simulink model "Integrated_controlled_system"  (R2020a)
settings: Solver=VariableStepAuto  StartTime=0.0  StopTime=simStopTime  RelTol=1e-3
PostLoadFcn:
  | helperLFSetUp
values from neighbouring files (symbols this model uses):
  lr = 1.67    [LateralDynamicsCT05.m]    (also in controller_setup05.m; helperLFSetUp.m)
  m = 2272    [LateralDynamicsCT05.m]    (also in controller_setup05.m; helperLFSetUp.m)
  tau = 0.5    [helperLFSetUp.m]
  Tfault = 1    [helperLFSetUp.m]
  Ts = 0.1    [controller_setup05.m]    (also in helperLFSetUp.m)
  v_set = egoCar.v0    [helperLFSetUp.m]
undefined symbols (not defined in the file or in its folder): Curvature, CurvatureDerivative, driving, HeadingAngle, LateralOffset, Left, Right, Strength
libraries: drivingscenarioandsensors x5, autolibshared x1
CloseFcn:
  | helperLFCleanUp
settings Model: NumberOfSteps=10  Creator=The MathWorks, Inc.  LastModifiedBy=dekunw
settings DataIOCC: ReturnWorkspaceOutputs=off
settings DebuggingCC: ParameterPrecisionLossMsg=none  PregeneratedLibrarySubsystemCodeDiagnostic=none  ArithmeticOperatorsInVariantConditions=warning
settings HardwareCC: ProdLongLongMode=on
settings SFSimCC: SimUseLocalCustomCode=off
settings RTWCC: GenerateReport=on  RTWUseLocalCustomCode=off  LaunchReport=on
settings ConfigComp: CovScope=ReferencedModels  CovIncludeTopModel=off  CovHtmlReporting=on

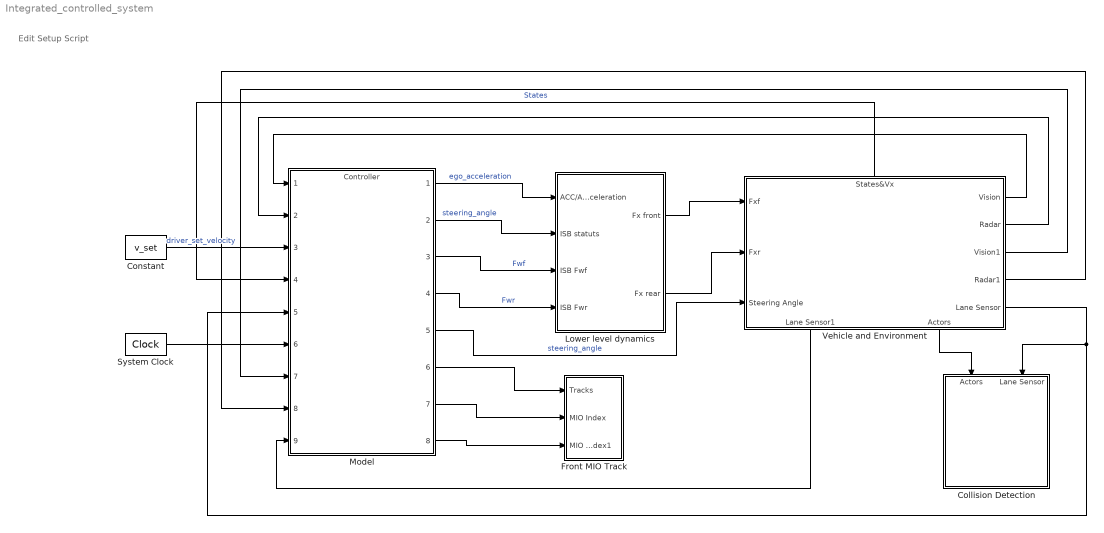
== system Integrated_controlled_system ==
  note: Edit Setup Script
  Collision Detection : Subsystem
  Constant : Constant  Value=v_set  SampleTime=Ts
  Front MIO Track : Subsystem
  Lower level dynamics : Subsystem
  Model : ModelReference  ModelNameDialog=Controller.slx  SimulationMode=Normal  ModelReferenceVersion=1.898
  System Clock : DigitalClock  SampleTime=Ts
  Vehicle and Environment : Subsystem
      settings: PortSchema="{\"entries\":[{\"content\":{\"sides\":[{\"content\":{\"connectorIds\":[\"In1\",\"In2\",\"In3\"]},\"type\":\"ConnectorPlacement.EquallySpacedRectSide\",\"uuid\":\"aa8441a5-2187-4ae6-b6bb-7d59e3966398\"},{\"content\":{\"connectorIds\":[\"Out1\",\"Out2\",\"Out3\",\"Out4\",\"Out5\"],\"side\":\"RIGHT\"},\"type\":\"ConnectorPlacement.EquallySpacedRectSide\",\"uuid\":\"2463696f-436c-42ea-9ab5-5fe7e39bf1c6\"},{\"content\":{\"connectorIds\":[\"Out8\"],\"side\":\"TOP\"},\"type\":\"ConnectorPlacement.EquallySpacedRectSide\",\"uuid\":\"ccb794f0-70b4-41ed-8f00-8d02b43a352e\"},{\"content\":{\"connectorIds\":[\"Out6\",\"Out7\"],\"side\":\"BOTTOM\"},\"type\":\"ConnectorPlacement.EquallySpacedRectSide\",\"uuid\":\"59090bb8-c4ce-44f0-8521-b892e1f18790\"}]},\"type\":\"ConnectorPlacement.EquallySpacedConnector\",\"uuid\":\"9ce6686a-073d-4311-a507-9f6c3ce68817\"}],\"packageUris\":[\"http://schema.mathworks.com/mf0/Connector/19700101\"],\"version\":\"1.0\"}"
  wires:
  Model/1 -> Lower level dynamics/1(ACC/AEB Acceleration)  "ego_acceleration"
  Model/5 -> Vehicle and Environment/3(Steering Angle)  "steering_angle"
  Constant/1 -> Model/3  "driver_set_velocity"
  Vehicle and Environment/8(States&Vx) -> Model/4  "States"
  Vehicle and Environment/5(Lane Sensor) -> Model/5, Collision Detection/2(Lane Sensor)
  Vehicle and Environment/2(Radar) -> Model/2
  Vehicle and Environment/1(Vision) -> Model/1
  Vehicle and Environment/7(Actors) -> Collision Detection/1(Actors)
  System Clock/1 -> Model/6
  Lower level dynamics/1(Fx front) -> Vehicle and Environment/1(Fxf)
  Lower level dynamics/2(Fx rear) -> Vehicle and Environment/2(Fxr)
  Model/2 -> Lower level dynamics/2(ISB statuts)  "steering_angle"
  Model/3 -> Lower level dynamics/3(ISB Fwf)  "Fwf"
  Model/4 -> Lower level dynamics/4(ISB Fwr)  "Fwr"
  Vehicle and Environment/3(Vision1) -> Model/7
  Vehicle and Environment/4(Radar1) -> Model/8
  Vehicle and Environment/6(Lane Sensor1) -> Model/9
  Model/6 -> Front MIO Track/1(Tracks)
  Model/7 -> Front MIO Track/2(MIO Index)
  Model/8 -> Front MIO Track/3(MIO Track Index1)

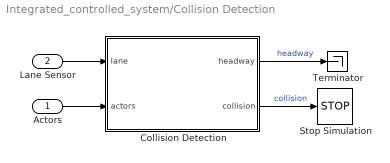
== system Integrated_controlled_system/Collision Detection ==
  Actors : Inport
  Lane Sensor : Inport  Port=2
  Collision Detection : MATLAB Function  TreatAsAtomicUnit=on
  Stop Simulation : Stop
  Terminator : Terminator
  wires:
  Collision Detection/2(collision) -> Stop Simulation/1  "collision"
  Actors/1 -> Collision Detection/2(actors)
  Lane Sensor/1 -> Collision Detection/1(lane)
  Collision Detection/1(headway) -> Terminator/1  "headway"

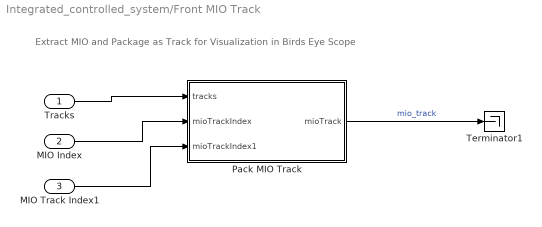
== system Integrated_controlled_system/Front MIO Track ==
  note: Extract MIO and Package as Track for Visualization in Birds Eye Scope
  Tracks : Inport
  MIO Index : Inport  Port=2
  MIO Track Index1 : Inport  Port=3
  Pack MIO Track : MATLAB Function  TreatAsAtomicUnit=on
  Terminator1 : Terminator
  wires:
  Tracks/1 -> Pack MIO Track/1(tracks)
  Pack MIO Track/1(mioTrack) -> Terminator1/1  "mio_track"
  MIO Index/1 -> Pack MIO Track/2(mioTrackIndex)
  MIO Track Index1/1 -> Pack MIO Track/3(mioTrackIndex1)

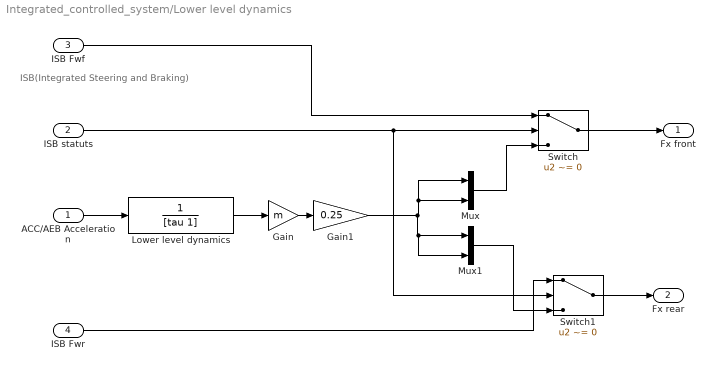
== system Integrated_controlled_system/Lower level dynamics ==
  note: ISB(Integrated Steering and Braking)
  ACC/AEB Acceleration : Inport
  ISB statuts : Inport  Port=2
  ISB Fwf : Inport  Port=3
  ISB Fwr : Inport  Port=4
  Gain : Gain  Gain=m
  Gain1 : Gain  Gain=0.25
  Lower level dynamics : TransferFcn  Denominator=[tau 1]
  Mux : Mux  Inputs=2
  Mux1 : Mux  Inputs=2
  Switch : Switch  Criteria=u2 ~= 0
  Switch1 : Switch  Criteria=u2 ~= 0
  Fx front : Outport  VectorParamsAs1DForOutWhenUnconnected=off
  Fx rear : Outport  Port=2  VectorParamsAs1DForOutWhenUnconnected=off
  wires:
  Gain/1 -> Gain1/1
  ACC/AEB Acceleration/1 -> Lower level dynamics/1
  Lower level dynamics/1 -> Gain/1
  Mux/1 -> Switch/3
  Mux1/1 -> Switch1/3
  Gain1/1 -> Mux1/2, Mux1/1, Mux/2, Mux/1
  ISB statuts/1 -> Switch1/2, Switch/2
  Switch/1 -> Fx front/1
  Switch1/1 -> Fx rear/1
  ISB Fwr/1 -> Switch1/1
  ISB Fwf/1 -> Switch/1

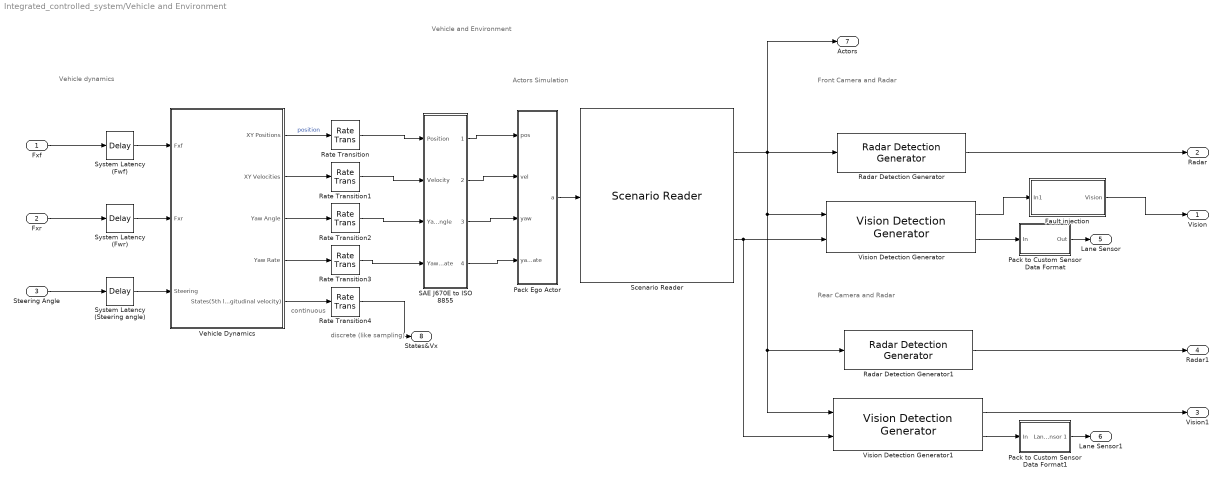
== system Integrated_controlled_system/Vehicle and Environment ==
  note: Front Camera and Radar
  note: continuous
  note: Vehicle dynamics
  note: Vehicle and Environment
  note: discrete (like sampling)
  note: Actors Simulation
  note: Rear Camera and Radar
  Fxf : Inport  Unit=N
  Fxr : Inport  Port=2  Unit=N
  Steering Angle : Inport  Port=3  Unit=rad
  Fault injection : Subsystem
  Pack Ego Actor : MATLAB Function  TreatAsAtomicUnit=on
  Pack to Custom Sensor Data Format : Subsystem
  Pack to Custom Sensor Data Format1 : Subsystem
  Radar Detection Generator : drivingscenarioandsensors/Radar Detection Generator  SensorIndex=2  UpdateInterval=0.1  SensorLocation=[ 3.7, 0 ]  Height=0.2  Yaw=0  Pitch=0  Roll=0  BusNameSource=Property  BusName=BusRadar  MaxNumDetectionsSource=Property  MaxNumDetections=50  DetectionCoordinates=Ego Cartesian  SimulateUsing=Interpreted execution  AzimuthResolution=4  ElevationResolution=10  RangeResolution=2.5  RangeRateResolution=0.5  AzimuthBiasFraction=0.1  ElevationBiasFraction=0.1  RangeBiasFraction=0.05  RangeRateBiasFraction=0.05  FieldOfView=[ 20, 5 ]  MaxRange=174  RangeRateLimits=[ -100, 100 ]  DetectionProbability=0.9  FalseAlarmRate=1e-6  ReferenceRange=100  ReferenceRCS=0  HasElevation=off  HasRangeRate=on  HasNoise=on  HasFalseAlarms=on  HasOcclusion=on  InitialSeedSource=Repeatable  InitialSeed=0  UsedSeed=driving.internal.SimulinkUtilities.seedManager(gcb)  ActorProfilesSource=MATLAB expression  ActorProfilesParameters=driving.internal.ActorProfilesRadarParameters  ActorProfilesExpression=actor_Profiles
      settings: SourceProductBaseCode=DR
  Radar Detection Generator1 : drivingscenarioandsensors/Radar Detection Generator  SensorIndex=4  UpdateInterval=0.1  SensorLocation=[ -1, 0 ]  Height=0.2  Yaw=180  Pitch=0  Roll=0  BusNameSource=Property  BusName=BusRadar  MaxNumDetectionsSource=Property  MaxNumDetections=50  DetectionCoordinates=Ego Cartesian  SimulateUsing=Interpreted execution  AzimuthResolution=4  ElevationResolution=10  RangeResolution=2.5  RangeRateResolution=0.5  AzimuthBiasFraction=0.1  ElevationBiasFraction=0.1  RangeBiasFraction=0.05  RangeRateBiasFraction=0.05  FieldOfView=[ 20, 5 ]  MaxRange=174  RangeRateLimits=[ -100, 100 ]  DetectionProbability=0.9  FalseAlarmRate=1e-6  ReferenceRange=100  ReferenceRCS=0  HasElevation=off  HasRangeRate=on  HasNoise=on  HasFalseAlarms=on  HasOcclusion=on  InitialSeedSource=Repeatable  InitialSeed=0  UsedSeed=driving.internal.SimulinkUtilities.seedManager(gcb)  ActorProfilesSource=MATLAB expression  ActorProfilesParameters=driving.internal.ActorProfilesRadarParameters  ActorProfilesExpression=actor_Profiles
      settings: SourceProductBaseCode=DR
  Rate Transition{,1..4} (5 alike) : RateTransition  OutPortSampleTime=Ts
  SAE J670E to ISO 8855 : Subsystem
  Scenario Reader : drivingscenarioandsensors/Scenario Reader  ScenarioSource=From file  ScenarioFileName=AEB_wdk.mat  ScenarioVariableName=scenario  OutputCoordinateSystem=Vehicle coordinates  EgoVehicleSource=Input port  OrientVehiclesOnRoad=off  EgoVehicleActorID=1  OutputEgoVehiclePose=off  SampleTime=0.1  LaneBoundaryOutput=Ego vehicle lane boundaries  LaneBoundaryDistance=0:0.5:60  LaneBoundaryLocation=Inner edge of lane markings  BusNameSource=Auto  BusName=BusActors  BusName2Source=Auto  BusName2=BusLaneBoundaries  BusName3Source=Auto  BusName3=BusEgoActor  ShowCoordinateLabels=on  SimulateUsing=Interpreted execution
  System Latency (Fwf) : TransportDelay  DelayTime=Ts
  System Latency (Fwr) : TransportDelay  DelayTime=Ts
  System Latency (Steering angle) : TransportDelay  DelayTime=Ts
  Vehicle Dynamics : Subsystem  VariantControl=Variant2
  Vision Detection Generator : drivingscenarioandsensors/Vision Detection Generator  SensorIndex=1  DetectorOutput=Lanes and objects  UpdateInterval=0.1  LaneUpdateInterval=0.1  SensorLocation=[ 1.9, 0 ]  Height=1.1  Yaw=0  Pitch=1  Roll=0  BusNameSource=Property  BusName=BusVision  BusName2Source=Property  BusName2=BusLanes  MaxNumDetectionsSource=Property  MaxNumDetections=20  MaxNumLanesSource=Property  MaxNumLanes=2  DetectionCoordinates=Ego Cartesian  SimulateUsing=Interpreted execution  MaxRange=150  BoundingBoxAccuracy=5  ProcessNoiseIntensity=5  MaxSpeed=50  MaxAllowedOcclusion=0.5  MinObjectImageSize=[ 10, 10 ]  DetectionProbability=0.9  FalsePositivesPerImage=0.1  MinLaneImageSize=[ 20, 3 ]  LaneBoundaryAccuracy=3  HasNoise=on  InitialSeedSource=Repeatable  InitialSeed=0  UsedSeed=driving.internal.SimulinkUtilities.seedManager(gcb)  ActorProfilesSource=MATLAB expression  ActorProfilesParameters=driving.internal.ActorProfilesParameters  ActorProfilesExpression=actor_Profiles  Intrinsics=driving.internal.cameraIntrinsics('FocalLength',[ 800,800 ])
  Vision Detection Generator1 : drivingscenarioandsensors/Vision Detection Generator  SensorIndex=3  DetectorOutput=Lanes and objects  UpdateInterval=0.1  LaneUpdateInterval=0.1  SensorLocation=[ 0.5, 0 ]  Height=1.1  Yaw=180  Pitch=1  Roll=0  BusNameSource=Property  BusName=BusVision  BusName2Source=Property  BusName2=BusLanes  MaxNumDetectionsSource=Property  MaxNumDetections=20  MaxNumLanesSource=Property  MaxNumLanes=2  DetectionCoordinates=Ego Cartesian  SimulateUsing=Interpreted execution  MaxRange=150  BoundingBoxAccuracy=5  ProcessNoiseIntensity=5  MaxSpeed=50  MaxAllowedOcclusion=0.5  MinObjectImageSize=[ 10, 10 ]  DetectionProbability=0.9  FalsePositivesPerImage=0.1  MinLaneImageSize=[ 20, 3 ]  LaneBoundaryAccuracy=3  HasNoise=on  InitialSeedSource=Repeatable  InitialSeed=0  UsedSeed=driving.internal.SimulinkUtilities.seedManager(gcb)  ActorProfilesSource=MATLAB expression  ActorProfilesParameters=driving.internal.ActorProfilesParameters  ActorProfilesExpression=actor_Profiles  Intrinsics=driving.internal.cameraIntrinsics('FocalLength',[ 800,800 ])
  Vision : Outport  VectorParamsAs1DForOutWhenUnconnected=off
  Radar : Outport  Port=2  VectorParamsAs1DForOutWhenUnconnected=off
  Vision1 : Outport  Port=3  VectorParamsAs1DForOutWhenUnconnected=off
  Radar1 : Outport  Port=4  VectorParamsAs1DForOutWhenUnconnected=off
  Lane Sensor : Outport  Port=5  VectorParamsAs1DForOutWhenUnconnected=off
  Lane Sensor1 : Outport  Port=6  VectorParamsAs1DForOutWhenUnconnected=off
  Actors : Outport  Port=7  VectorParamsAs1DForOutWhenUnconnected=off
  States&Vx : Outport  Port=8  VectorParamsAs1DForOutWhenUnconnected=off
  wires:
  Scenario Reader/1 -> Actors/1, Radar Detection Generator/1, Vision Detection Generator/1, Vision Detection Generator1/1, Radar Detection Generator1/1
  Vehicle Dynamics/2(XY Velocities) -> Rate Transition1/1
  Vehicle Dynamics/3(Yaw Angle) -> Rate Transition2/1
  Vehicle Dynamics/4(Yaw Rate) -> Rate Transition3/1
  Vehicle Dynamics/1(XY Positions) -> Rate Transition/1  "position"
  Vision Detection Generator/2 -> Pack to Custom Sensor Data Format/1(In)
  Pack to Custom Sensor Data Format/1(Out) -> Lane Sensor/1
  Rate Transition4/1 -> States&Vx/1
  Vehicle Dynamics/5(States(5th longitudinal velocity)) -> Rate Transition4/1
  Scenario Reader/2 -> Vision Detection Generator1/2, Vision Detection Generator/2
  Pack Ego Actor/1(a) -> Scenario Reader/1
  Steering Angle/1 -> System Latency (Steering angle)/1
  System Latency (Steering angle)/1 -> Vehicle Dynamics/3(Steering)
  Fxf/1 -> System Latency (Fwf)/1
  System Latency (Fwf)/1 -> Vehicle Dynamics/1(Fxf)
  Fxr/1 -> System Latency (Fwr)/1
  System Latency (Fwr)/1 -> Vehicle Dynamics/2(Fxr)
  Rate Transition/1 -> SAE J670E to ISO 8855/1(Position)
  Rate Transition1/1 -> SAE J670E to ISO 8855/2(Velocity)
  Rate Transition2/1 -> SAE J670E to ISO 8855/3(Yaw Angle)
  Rate Transition3/1 -> SAE J670E to ISO 8855/4(Yaw Rate)
  SAE J670E to ISO 8855/1(1) -> Pack Ego Actor/1(pos)
  SAE J670E to ISO 8855/2(2) -> Pack Ego Actor/2(vel)
  SAE J670E to ISO 8855/3(3) -> Pack Ego Actor/3(yaw)
  SAE J670E to ISO 8855/4(4) -> Pack Ego Actor/4(yawRate)
  Radar Detection Generator/1 -> Radar/1
  Vision Detection Generator/1 -> Fault injection/1(In1)
  Vision Detection Generator1/2 -> Pack to Custom Sensor Data Format1/1(In)
  Vision Detection Generator1/1 -> Vision1/1
  Radar Detection Generator1/1 -> Radar1/1
  Pack to Custom Sensor Data Format1/1(Lane Sensor 1) -> Lane Sensor1/1
  Fault injection/1(Vision) -> Vision/1

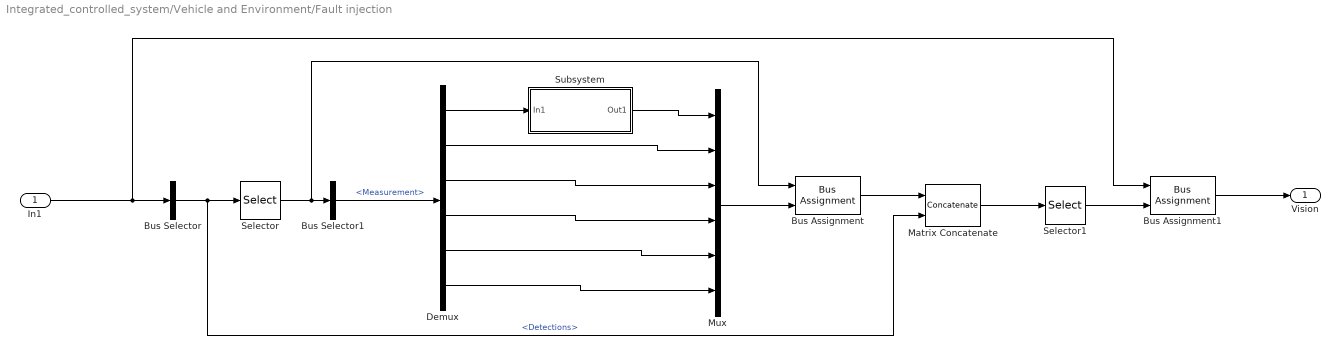
== system Integrated_controlled_system/Vehicle and Environment/Fault injection ==
  In1 : Inport
  Bus Assignment : BusAssignment  AssignedSignals=Measurement
  Bus Assignment1 : BusAssignment  AssignedSignals=Detections
  Bus Selector : BusSelector  OutputSignals=Detections
  Bus Selector1 : BusSelector  OutputSignals=Measurement
  Demux : Demux  Outputs=6
  Matrix Concatenate : Concatenate  Mode=Multidimensional array
  Mux : Mux  Inputs=6
  Selector : Selector  InputPortWidth=20  IndexOptions=Index vector (dialog)  Indices=1  OutputSizes=1
  Selector1 : Selector  InputPortWidth=21  IndexOptions=Index vector (dialog)  Indices=[1 3 4 5 6 7 8 9 10 11 12 13 14 15 16 17 18 19 20 21]  OutputSizes=1
  Subsystem : Subsystem
  Vision : Outport
  wires:
  Bus Selector/1 -> Matrix Concatenate/2, Selector/1  "<Detections>"
  Demux/2 -> Mux/2
  Subsystem/1(Out1) -> Mux/1
  Selector/1 -> Bus Assignment/1, Bus Selector1/1
  Selector1/1 -> Bus Assignment1/2
  Bus Assignment1/1 -> Vision/1
  Demux/1 -> Subsystem/1(In1)
  Bus Selector1/1 -> Demux/1  "<Measurement>"
  In1/1 -> Bus Assignment1/1, Bus Selector/1
  Matrix Concatenate/1 -> Selector1/1
  Bus Assignment/1 -> Matrix Concatenate/1
  Demux/6 -> Mux/6
  Mux/1 -> Bus Assignment/2
  Demux/4 -> Mux/4
  Demux/5 -> Mux/5
  Demux/3 -> Mux/3

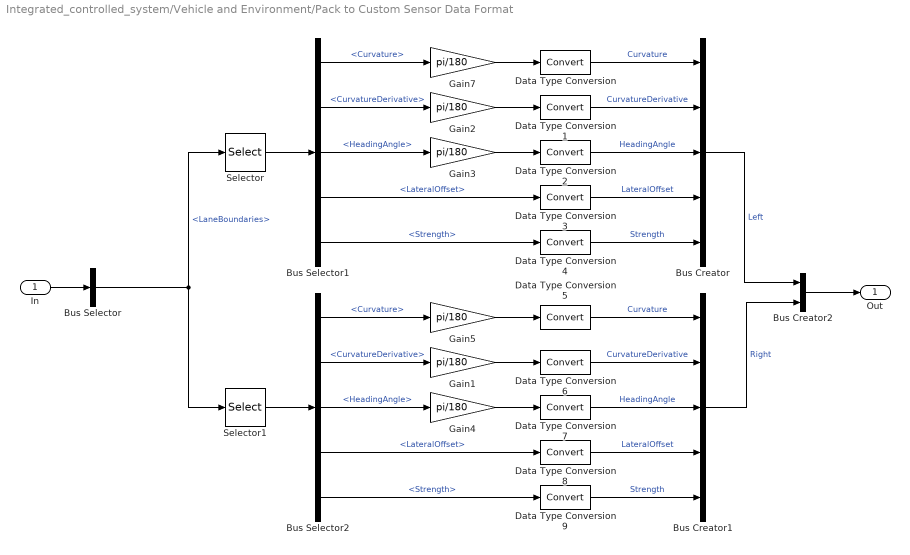
== system Integrated_controlled_system/Vehicle and Environment/Pack to Custom Sensor Data Format ==
  In : Inport
  Bus Creator : BusCreator  Inputs=Curvature,CurvatureDerivative,HeadingAngle,LateralOffset,Strength  OutDataTypeStr=Bus: LaneSensorBoundaries
  Bus Creator1 : BusCreator  Inputs=Curvature,CurvatureDerivative,HeadingAngle,LateralOffset,Strength  OutDataTypeStr=Bus: LaneSensorBoundaries
  Bus Creator2 : BusCreator  Inputs=Left,Right  OutDataTypeStr=Bus: LaneSensor
  Bus Selector : BusSelector  OutputSignals=LaneBoundaries
  Bus Selector1 : BusSelector  OutputSignals=Curvature,CurvatureDerivative,HeadingAngle,LateralOffset,Strength
  Bus Selector2 : BusSelector  OutputSignals=Curvature,CurvatureDerivative,HeadingAngle,LateralOffset,Strength
  Data Type Conversion{,1..9} (10 alike) : DataTypeConversion
  Gain{1..5,7} (6 alike) : Gain  Gain=pi/180
  Selector : Selector  InputPortWidth=2  IndexOptions=Index vector (dialog)  Indices=1  OutputSizes=1
  Selector1 : Selector  InputPortWidth=2  IndexOptions=Index vector (dialog)  Indices=2  OutputSizes=1
  Out : Outport  VectorParamsAs1DForOutWhenUnconnected=off
  wires:
  In/1 -> Bus Selector/1
  Bus Selector/1 -> Selector/1, Selector1/1  "<LaneBoundaries>"
  Selector/1 -> Bus Selector1/1
  Bus Selector1/2 -> Gain2/1  "<CurvatureDerivative>"
  Bus Selector1/1 -> Gain7/1  "<Curvature>"
  Bus Selector1/3 -> Gain3/1  "<HeadingAngle>"
  Gain7/1 -> Data Type Conversion/1
  Gain2/1 -> Data Type Conversion1/1
  Gain3/1 -> Data Type Conversion2/1
  Bus Selector1/4 -> Data Type Conversion3/1  "<LateralOffset>"
  Bus Selector1/5 -> Data Type Conversion4/1  "<Strength>"
  Data Type Conversion/1 -> Bus Creator/1  "Curvature"
  Data Type Conversion1/1 -> Bus Creator/2  "CurvatureDerivative"
  Data Type Conversion2/1 -> Bus Creator/3  "HeadingAngle"
  Data Type Conversion3/1 -> Bus Creator/4  "LateralOffset"
  Data Type Conversion4/1 -> Bus Creator/5  "Strength"
  Data Type Conversion9/1 -> Bus Creator1/5  "Strength"
  Data Type Conversion6/1 -> Bus Creator1/2  "CurvatureDerivative"
  Data Type Conversion7/1 -> Bus Creator1/3  "HeadingAngle"
  Data Type Conversion8/1 -> Bus Creator1/4  "LateralOffset"
  Data Type Conversion5/1 -> Bus Creator1/1  "Curvature"
  Bus Selector2/1 -> Gain5/1  "<Curvature>"
  Selector1/1 -> Bus Selector2/1
  Bus Selector2/4 -> Data Type Conversion8/1  "<LateralOffset>"
  Bus Selector2/5 -> Data Type Conversion9/1  "<Strength>"
  Bus Selector2/2 -> Gain1/1  "<CurvatureDerivative>"
  Gain4/1 -> Data Type Conversion7/1
  Gain5/1 -> Data Type Conversion5/1
  Gain1/1 -> Data Type Conversion6/1
  Bus Selector2/3 -> Gain4/1  "<HeadingAngle>"
  Bus Creator2/1 -> Out/1
  Bus Creator/1 -> Bus Creator2/1  "Left"
  Bus Creator1/1 -> Bus Creator2/2  "Right"

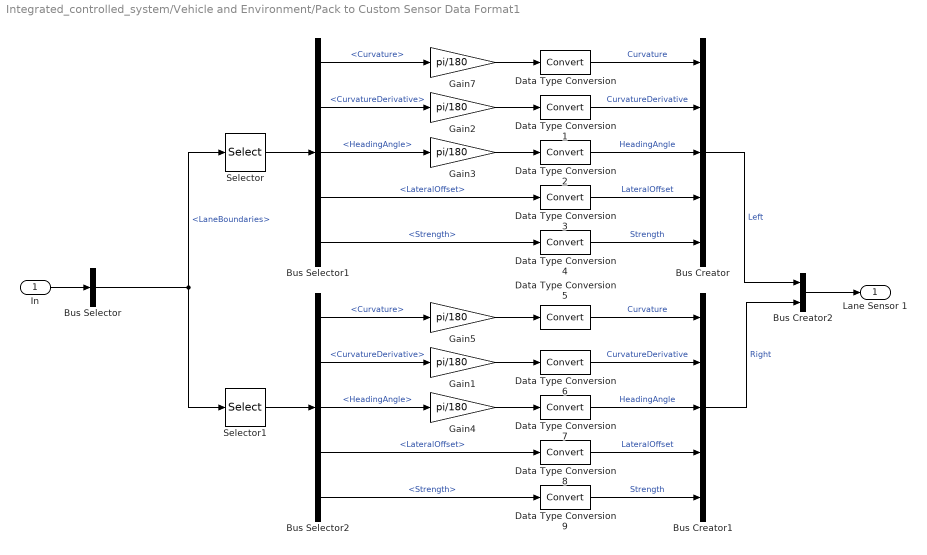
== system Integrated_controlled_system/Vehicle and Environment/Pack to Custom Sensor Data Format1 ==
  In : Inport
  Bus Creator : BusCreator  Inputs=Curvature,CurvatureDerivative,HeadingAngle,LateralOffset,Strength  OutDataTypeStr=Bus: LaneSensorBoundaries
  Bus Creator1 : BusCreator  Inputs=Curvature,CurvatureDerivative,HeadingAngle,LateralOffset,Strength  OutDataTypeStr=Bus: LaneSensorBoundaries
  Bus Creator2 : BusCreator  Inputs=Left,Right  OutDataTypeStr=Bus: LaneSensor
  Bus Selector : BusSelector  OutputSignals=LaneBoundaries
  Bus Selector1 : BusSelector  OutputSignals=Curvature,CurvatureDerivative,HeadingAngle,LateralOffset,Strength
  Bus Selector2 : BusSelector  OutputSignals=Curvature,CurvatureDerivative,HeadingAngle,LateralOffset,Strength
  Data Type Conversion{,1..9} (10 alike) : DataTypeConversion
  Gain{1..5,7} (6 alike) : Gain  Gain=pi/180
  Selector : Selector  InputPortWidth=2  IndexOptions=Index vector (dialog)  Indices=1  OutputSizes=1
  Selector1 : Selector  InputPortWidth=2  IndexOptions=Index vector (dialog)  Indices=2  OutputSizes=1
  Lane Sensor 1 : Outport  VectorParamsAs1DForOutWhenUnconnected=off
  wires:
  In/1 -> Bus Selector/1
  Bus Selector/1 -> Selector/1, Selector1/1  "<LaneBoundaries>"
  Selector/1 -> Bus Selector1/1
  Bus Selector1/2 -> Gain2/1  "<CurvatureDerivative>"
  Bus Selector1/1 -> Gain7/1  "<Curvature>"
  Bus Selector1/3 -> Gain3/1  "<HeadingAngle>"
  Gain7/1 -> Data Type Conversion/1
  Gain2/1 -> Data Type Conversion1/1
  Gain3/1 -> Data Type Conversion2/1
  Bus Selector1/4 -> Data Type Conversion3/1  "<LateralOffset>"
  Bus Selector1/5 -> Data Type Conversion4/1  "<Strength>"
  Data Type Conversion/1 -> Bus Creator/1  "Curvature"
  Data Type Conversion1/1 -> Bus Creator/2  "CurvatureDerivative"
  Data Type Conversion2/1 -> Bus Creator/3  "HeadingAngle"
  Data Type Conversion3/1 -> Bus Creator/4  "LateralOffset"
  Data Type Conversion4/1 -> Bus Creator/5  "Strength"
  Data Type Conversion9/1 -> Bus Creator1/5  "Strength"
  Data Type Conversion6/1 -> Bus Creator1/2  "CurvatureDerivative"
  Data Type Conversion7/1 -> Bus Creator1/3  "HeadingAngle"
  Data Type Conversion8/1 -> Bus Creator1/4  "LateralOffset"
  Data Type Conversion5/1 -> Bus Creator1/1  "Curvature"
  Bus Selector2/1 -> Gain5/1  "<Curvature>"
  Selector1/1 -> Bus Selector2/1
  Bus Selector2/4 -> Data Type Conversion8/1  "<LateralOffset>"
  Bus Selector2/5 -> Data Type Conversion9/1  "<Strength>"
  Bus Selector2/2 -> Gain1/1  "<CurvatureDerivative>"
  Gain4/1 -> Data Type Conversion7/1
  Gain5/1 -> Data Type Conversion5/1
  Gain1/1 -> Data Type Conversion6/1
  Bus Selector2/3 -> Gain4/1  "<HeadingAngle>"
  Bus Creator2/1 -> Lane Sensor 1/1
  Bus Creator/1 -> Bus Creator2/1  "Left"
  Bus Creator1/1 -> Bus Creator2/2  "Right"

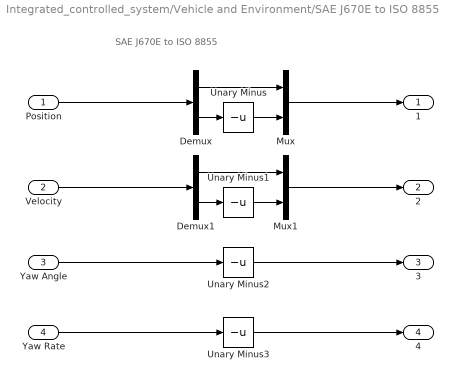
== system Integrated_controlled_system/Vehicle and Environment/SAE J670E to ISO 8855 ==
  note: SAE J670E to ISO 8855
  Position : Inport  Unit=m
  Velocity : Inport  Port=2  Unit=m/s
  Yaw Angle : Inport  Port=3  Unit=deg
  Yaw Rate : Inport  Port=4  Unit=deg/s
  Demux : Demux  Outputs=2
  Demux1 : Demux  Outputs=2
  Mux : Mux  Inputs=2
  Mux1 : Mux  Inputs=2
  Unary Minus{,1..3} (4 alike) : UnaryMinus
  1 : Outport  VectorParamsAs1DForOutWhenUnconnected=off
  2 : Outport  Port=2  VectorParamsAs1DForOutWhenUnconnected=off
  3 : Outport  Port=3  VectorParamsAs1DForOutWhenUnconnected=off
  4 : Outport  Port=4  VectorParamsAs1DForOutWhenUnconnected=off
  wires:
  Yaw Rate/1 -> Unary Minus3/1
  Yaw Angle/1 -> Unary Minus2/1
  Demux/1 -> Mux/1
  Demux/2 -> Unary Minus/1
  Unary Minus/1 -> Mux/2
  Unary Minus1/1 -> Mux1/2
  Demux1/2 -> Unary Minus1/1
  Demux1/1 -> Mux1/1
  Mux1/1 -> 2/1
  Mux/1 -> 1/1
  Position/1 -> Demux/1
  Velocity/1 -> Demux1/1
  Unary Minus2/1 -> 3/1
  Unary Minus3/1 -> 4/1

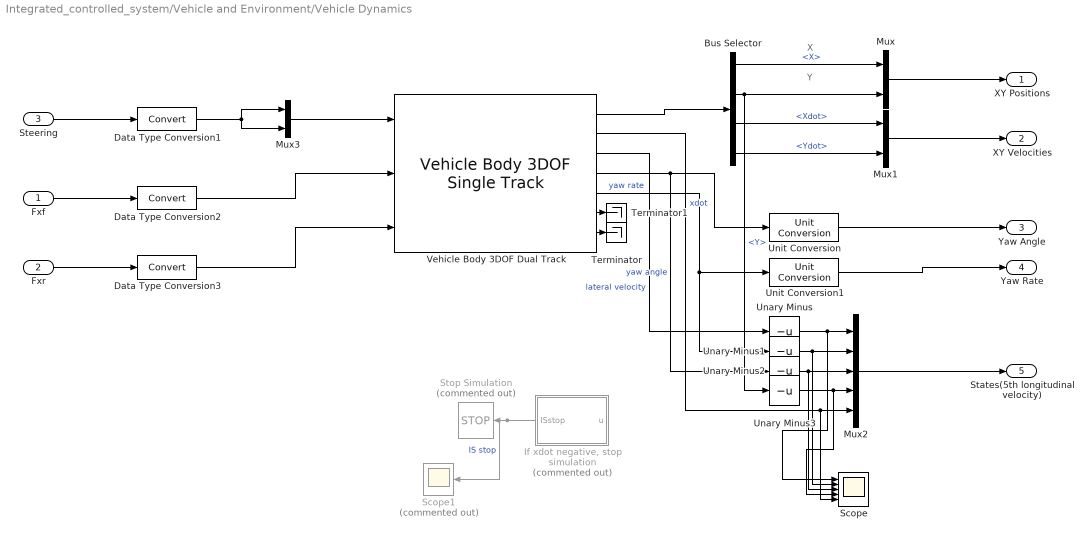
== system Integrated_controlled_system/Vehicle and Environment/Vehicle Dynamics ==
  note: Y
  note: X
  Fxf : Inport  Unit=N
  Fxr : Inport  Port=2  Unit=N
  Steering : Inport  Port=3  Unit=rad
  Bus Selector : BusSelector  OutputSignals=InertFrm.Cg.Disp.X,InertFrm.Cg.Disp.Y,InertFrm.Cg.Vel.Xdot,InertFrm.Cg.Vel.Ydot
  Data Type Conversion1 : DataTypeConversion
  Data Type Conversion2 : DataTypeConversion
  Data Type Conversion3 : DataTypeConversion
  "If xdot negative, stop simulation" : MATLAB Function  Commented=on  TreatAsAtomicUnit=on
  Mux : Mux  Inputs=2
  Mux1 : Mux  Inputs=2
  Mux2 : Mux  Inputs=5
  Mux3 : Mux  Inputs=2
  Scope : Scope  NumInputPorts=5
  Scope1 : Scope  Commented=on
  Stop Simulation : Stop  Commented=on
  Terminator : Terminator
  Terminator1 : Terminator
  Unary Minus{,1..3} (4 alike) : UnaryMinus
  Unit Conversion : UnitConversion  OutputType=Inherit: Inherit via back propagation
  Unit Conversion1 : UnitConversion  OutputType=Inherit: Inherit via back propagation
  Vehicle Body 3DOF Dual Track : autolibshared/Vehicle Body 3DOF Single Track  trackMode=Dual  inputMode=External longitudinal forces  frontSteerMode=on  rearSteerMode=off  windMode=off  muMode=off  extFMode=off  extMMode=off  extXo=off  extpsio=off  extxdoto=off  extro=off  extYo=off  extTamb=off  extydoto=off  aMode=2  NF=2  NR=2  m=m  a=lf  b=lr  h=0.35  X_o=x0_ego  xdot_o=v0_ego  CalphaMode=off  sigmaMode=on  d=0  w=[1.4,1.4]  Cy_f=Cf  Cy_r=Cr  sigma_f=.1  sigma_r=.1  alpha_f_brk=[-.1 .1]  Cy_f_data=[-9e3 9e3]  alpha_r_brk=[-.1 .1]  Cy_r_data=[-9e3 9e3]  Y_o=y0_ego  ydot_o=0  Izz=Iz  psi_o=yaw0_ego  r_o=0  Af=2  Cd=.3  Cl=.1  Cpm=.1  beta_w=[0:0.01:0.3]  Cs=[0:0.03:0.9]  Cym=[0:0.01:0.3]  Pabs=101325  Tair=273  g=9.81  mu=miu  xdot_tol=.01  Fznom=5000  Fxtire_sat=7e4  Fytire_sat=7e4  longOff=0  latOff=0  vertOff=0  wrapAng=off
      settings: SourceProductBaseCode=PW,MT,VE,VP
  XY Positions : Outport  Unit=m  VectorParamsAs1DForOutWhenUnconnected=off
  XY Velocities : Outport  Port=2  Unit=m/s  VectorParamsAs1DForOutWhenUnconnected=off
  Yaw Angle : Outport  Port=3  Unit=deg  VectorParamsAs1DForOutWhenUnconnected=off
  Yaw Rate : Outport  Port=4  Unit=degree/s  VectorParamsAs1DForOutWhenUnconnected=off
  States(5th longitudinal velocity) : Outport  Port=5  VectorParamsAs1DForOutWhenUnconnected=off
  wires:
  Fxf/1 -> Data Type Conversion2/1
  Data Type Conversion1/1 -> Mux3/2, Mux3/1
  Steering/1 -> Data Type Conversion1/1
  Bus Selector/1 -> Mux/1  "<X>"
  Unit Conversion/1 -> Yaw Angle/1
  Vehicle Body 3DOF Dual Track/5 -> Unary Minus1/1, Unit Conversion1/1  "yaw rate"
  Bus Selector/4 -> Mux1/2  "<Ydot>"
  Vehicle Body 3DOF Dual Track/4 -> Unary Minus2/1, Unit Conversion/1  "yaw angle"
  Bus Selector/2 -> Unary Minus3/1, Mux/2  "<Y>"
  Bus Selector/3 -> Mux1/1  "<Xdot>"
  Vehicle Body 3DOF Dual Track/1 -> Bus Selector/1
  Mux/1 -> XY Positions/1
  Mux1/1 -> XY Velocities/1
  Unit Conversion1/1 -> Yaw Rate/1
  Vehicle Body 3DOF Dual Track/6 -> Terminator1/1
  Vehicle Body 3DOF Dual Track/7 -> Terminator/1
  Vehicle Body 3DOF Dual Track/3 -> Unary Minus/1  "lateral velocity"
  Vehicle Body 3DOF Dual Track/2 -> Scope/5, Mux2/5  "xdot"
  Mux2/1 -> States(5th longitudinal velocity)/1
  Data Type Conversion2/1 -> Vehicle Body 3DOF Dual Track/2
  Mux3/1 -> Vehicle Body 3DOF Dual Track/1
  Fxr/1 -> Data Type Conversion3/1
  Data Type Conversion3/1 -> Vehicle Body 3DOF Dual Track/3
  Unary Minus/1 -> Scope/1, Mux2/1
  Unary Minus1/1 -> Scope/2, Mux2/2
  Unary Minus2/1 -> Scope/3, Mux2/3
  Unary Minus3/1 -> Scope/4, Mux2/4
  "If xdot negative, stop simulation"/1(ISstop) -> Scope1/1, Stop Simulation/1  "IS stop"

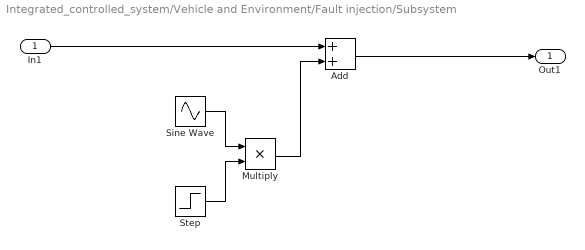
== system Integrated_controlled_system/Vehicle and Environment/Fault injection/Subsystem ==
  In1 : Inport
  Add : Sum
  Multiply : Product  Inputs=**
  Sine Wave : Sin  Frequency=pi  SampleTime=0.1
  Step : Step  Time=Tfault  SampleTime=0.1
  Out1 : Outport
  wires:
  In1/1 -> Add/1
  Sine Wave/1 -> Multiply/1
  Step/1 -> Multiply/2
  Multiply/1 -> Add/2
  Add/1 -> Out1/1

== matlab function Integrated_controlled_system/Collision Detection/Collision Detection ==
  data: lane input; headway output; actors input; collision output
function [headway,collision] = collisionDetect(lane, actors)

% If lane detection is not available, the ego car is assumed to be located
% in the middle of its lane. The lane width is assumed to be 3.6m, typical
% highway lane width.
laneWidth = 3.6;
halfLaneWidth = laneWidth/2;

% left lane
if lane.Left.Strength > 0.01
    lb = [lane.Left.CurvatureDerivative/6,...
        lane.Left.Curvature/2,...
        lane.Left.HeadingAngle,...
        lane.Left.LateralOffset];
else
    lb = single([0,0,0,halfLaneWidth]);
end

% right lane
if lane.Right.Strength > 0.01
    rb = [lane.Right.CurvatureDerivative/6,...
        lane.Right.Curvature/2,...
        lane.Right.HeadingAngle,...
        lane.Right.LateralOffset];
else
    rb = single([0,0,0,-halfLaneWidth]);    
end

dist = zeros(1,actors.NumActors);

for i = 1:actors.NumActors
    x = actors.Actors(i).Position(1);
    y = actors.Actors(i).Position(2);
    
    yleftLane  = polyval(lb,x);
    yrightLane = polyval(rb,x);
    
    if (yrightLane <= y) && (y <= yleftLane) % within lane boundary?
        dist(i) = hypot(x,y); 
    else
        dist(i) = 100;
    end       
end

headway = min(dist) - 4.7;  % headway from the lead vehicle's trailing surface to the ego vehicle's leading surface
if headway < 1.5
    collision = true; % collision detected
else
    collision = false;
end

== matlab function Integrated_controlled_system/Front MIO Track/Pack MIO Track ==
  data: tracks input; mioTrack output Bus: BusMultiObjectTracker1; mioTrackIndex input; mioTrackIndex1 input
function mioTrack = fcn(tracks, mioTrackIndex, mioTrackIndex1)
% Extract MIO track and package for visualization in Birds Eye Scope

mioTrack = tracks;

if mioTrackIndex > 0 && mioTrackIndex1 > 0
    % First track represents MIO
    mioTrack.NumTracks = 2;
    mioTrack.Tracks(1) = tracks.Tracks(mioTrackIndex);
    mioTrack.Tracks(2) = tracks.Tracks(mioTrackIndex1);
elseif mioTrackIndex > 0
    mioTrack.NumTracks = 1;
    mioTrack.Tracks(1) = tracks.Tracks(mioTrackIndex);
elseif mioTrackIndex1 > 0    
    mioTrack.NumTracks = 1;
    mioTrack.Tracks(1) = tracks.Tracks(mioTrackIndex1);
else
    % No valid MIO track
    mioTrack.NumTracks = 0;
end

== matlab function Integrated_controlled_system/Vehicle and Environment/Vehicle Dynamics/If xdot negative, stop simulation ==
  data: u input; ISstop output
function ISstop = fcn(u)
if u>0
    ISstop = false;
else
    ISstop = true;
end

== matlab function Integrated_controlled_system/Vehicle and Environment/Pack Ego Actor ==
  data: pos input; a output Bus: BusActors1Actors size=1; vel input; yaw input; yawRate input
function a = packEgo(pos,vel,yaw,yawRate)
% Pack ego information into a single ego actor bus
%
% Imoprtant note:
% Output is a bus of type BusActorsActors. This is the same bus used by the
% Scenario Reader to output an individual actor. If you change the
% output bus name of Scenario Reader change the output bus name here
% as well by clicking on 'Edit Data' in the menu above.

a = struct(...
    'ActorID',1,...
    'Position', [pos(1) pos(2) 0], ...
    'Velocity', [vel(1) vel(2) 0], ...
    'Roll', 0, ...
    'Pitch', 0, ...
    'Yaw', yaw, ...
    'AngularVelocity', [0 0 yawRate]);
